simulink model "model2_23_2"  (R2023b)
settings: Solver=FixedStepDiscrete  StartTime=0.0  StopTime=inf  RelTol=1e-3
model workspace (MAT data in the model file):
  simin = 10
libraries: commsequence2 x2, commchan3 x1, commrandsrc3 x1, simulink x1, commsink2 x1, dspsigops x1
settings Model: Creator=D.mon  LastModifiedBy=dymco

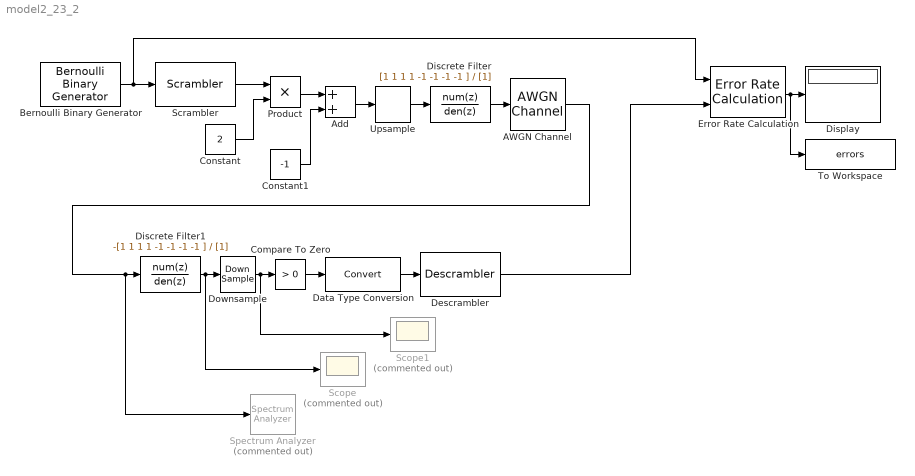
== system model2_23_2 ==
  AWGN Channel : commchan3/AWGN Channel  LegacyMode=off  NoiseMethod="Signal to noise ratio  (Es/No)"  noiseMode="Signal to noise ratio  (SNR)"  EbNo=10  EsNo=snr  SNR=snr  BitsPerSymbol=1  SignalPower=1  SamplesPerSymbol=8  SymbolPeriod=1  VarianceSource=Parameter  Variance=1  RandomStream=mt19937ar with seed  Seed=randi(100000)  SimulateUsing=Code generation
  Add : Sum
  Bernoulli Binary Generator : commrandsrc3/Bernoulli Binary Generator  ProbabilityOfZero=0.5  SeedSource=Auto  Seed=0  SampleTime=1  SamplesPerFrame=1  OutputDataType=double  SimulateUsing=Interpreted execution
  Compare To Zero : simulink/Logic and Bit Operations/Compare To Zero  relop=>  OutDataTypeStr=boolean
  Constant : Constant  Value=2
  Constant1 : Constant  Value=-1
  Data Type Conversion : DataTypeConversion  SaturateOnIntegerOverflow=off  RndMeth=Floor
  Descrambler : commsequence2/Descrambler  M=2  poly=[1 0 0 0 1 0 0 1]  iniStaSource=Dialog Parameter  ini_sta=0  resetViaPort=off
  Discrete Filter : DiscreteFilter  Numerator=[1 1 1 1 -1 -1 -1 -1 ]  Denominator=[1]
  Discrete Filter1 : DiscreteFilter  Numerator=-[1 1 1 1 -1 -1 -1 -1 ]  Denominator=[1]
  Display : Display
  Downsample : DownSample  N=8  phase=7  RateOptions=Allow multirate processing  AllowArbitraryFixedInput=on
  Error Rate Calculation : commsink2/Error Rate Calculation  N=1  st_delay=0  cp_mode=Entire frame  subframe=[]  PMode=Port  WsName=ErrorVec  RsMode2=off  stop=off  numErr=100  maxBits=1e6
  Product : Product
  Scope : Scope  Commented=on
  Scope1 : Scope  Commented=on
  Scrambler : commsequence2/Scrambler  M=2  poly=[1 0 0 0 1 0 0 1]  iniStaSource=Dialog Parameter  ini_sta=0  resetViaPort=off
  Spectrum Analyzer : SpectrumAnalyzer  Commented=on  WindowPosition=[1088.000000,198.000000,800.000000,500.000000,]  ScopeFrameLocation=window  Span=8  StartFrequency=-4  StopFrequency=4  YLimits=[-19.4034 30.2485]
  To Workspace : ToWorkspace  VariableName=errors  SampleTime=-1
      settings: MaxDataPoints=1  Save2DSignal=2-D array (concatenate along first dimension)
  Upsample : dspsigops/Upsample  FactorSource=Dialog parameter  N=8  Nmax=16  phase=0  InputProcessing=Columns as channels (frame based)  RateOptions=Allow multirate processing  ic=0  mode=Unused parameter value
  wires:
  Error Rate Calculation/1 -> To Workspace/1, Display/1
  Bernoulli Binary Generator/1 -> Scrambler/1, Error Rate Calculation/1
  Product/1 -> Add/1
  Constant/1 -> Product/2
  Constant1/1 -> Add/2
  Add/1 -> Upsample/1
  Compare To Zero/1 -> Data Type Conversion/1
  Data Type Conversion/1 -> Descrambler/1
  Upsample/1 -> Discrete Filter/1
  Discrete Filter/1 -> AWGN Channel/1
  Discrete Filter1/1 -> Scope/1, Downsample/1
  Downsample/1 -> Scope1/1, Compare To Zero/1
  AWGN Channel/1 -> Spectrum Analyzer/1, Discrete Filter1/1
  Scrambler/1 -> Product/1
  Descrambler/1 -> Error Rate Calculation/2
